simulink model "tempCyl4s"  (R2013a)
settings: Solver=ode15s  StartTime=0.0  StopTime=3  FixedStep=1e-3  RelTol=1e-5
values from neighbouring files (symbols this model uses):
  F0_ER = F_initial    [initHybrid.m]    (also in initMV.m; init_MVM.m)
  p0_AR = p_acool    [initHybrid.m]    (also in initMV.m; init_MVM.m)
  p0_ER = p_exh_init    [initHybrid.m]    (also in initMV.m; init_MVM.m)
  T0_AR = T_acool    [initHybrid.m]    (also in initMV.m; init_MVM.m)
  T0_ER = 800    [initHybrid.m]    (also in initMV.m; init_MVM.m)
  uGov = 0.2    [runTempCyl4S.m]
undefined symbols (not defined in the file): genset
libraries: EngineSystemSubmodelVer1_0 x6
settings Model: Creator=yum  LastModifiedBy=yum
settings DataIOCC: InspectSignalLogs=on

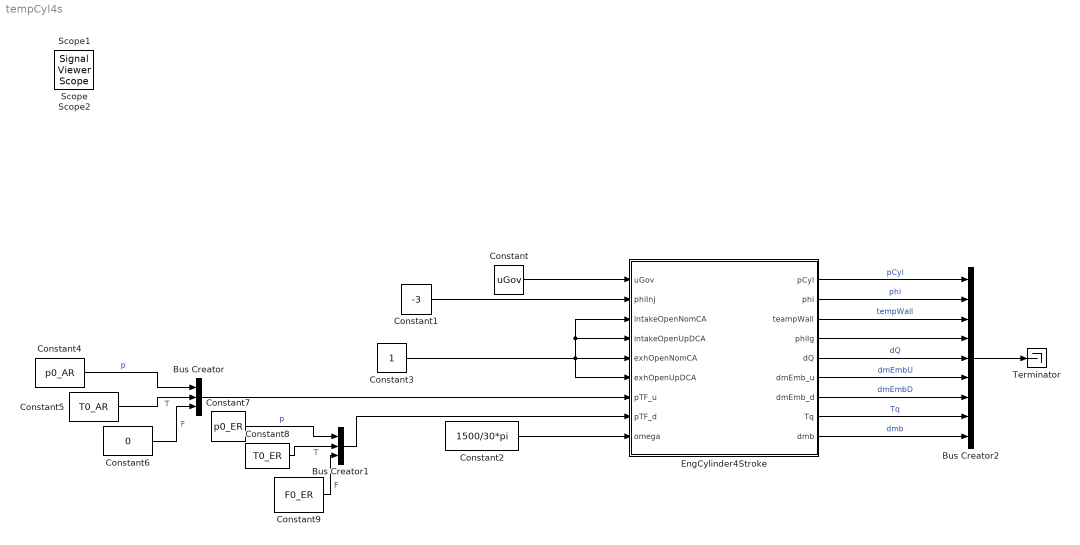
== system tempCyl4s ==
  Bus Creator : BusCreator  Inputs=3
  Bus Creator1 : BusCreator  Inputs=3
  Bus Creator2 : BusCreator  Inputs=9
  Constant : Constant  Value=uGov
  Constant1 : Constant  Value=-3
  Constant2 : Constant  Value=1500/30*pi
  Constant3 : Constant
  Constant4 : Constant  Value=p0_AR
  Constant5 : Constant  Value=T0_AR
  Constant6 : Constant  Value=0
  Constant7 : Constant  Value=p0_ER
  Constant8 : Constant  Value=T0_ER
  Constant9 : Constant  Value=F0_ER
  EngCylinder4Stroke : Subsystem  mask{fs=genset.eng.fs, nStroke=genset.eng.nStroke, hn=genset.eng.hn, nCyl=genset.eng.nCyl, iCyl=1, B=genset.eng.B, stroke=genset.eng.stroke, lambdaCrank=genset.eng.lambdaCrank, liftMaxIntake=genset.eng.intakeLiftMaxRef, DvIntake=genset.eng.intakeDV, betaIntake=genset.eng.intakeBeta, wIntake=genset.eng.intakeW, DpIntake=genset.eng.intakeDp, DsIntake=genset.eng.intakeDs, cAVVUpRef=genset.eng.cAVVUpRefIntake, cAVVDownRef=genset.eng.cAVVDownRefIntake, liftUpRef=genset.eng.liftUpRefIntake, liftDownRef=genset.eng.liftDownRefIntake, cAStartRef=genset.eng.startCARefIntake, dCALiftUp=genset.eng.dCALiftUpRefIntake, dCALiftDown=genset.eng.dCALiftDownIntake, dCALiftTopRef=genset.eng.dCALiftTopRefIntake, liftMaxExh=genset.eng.exhLiftMax, DvExh=genset.eng.exhDV, betaExh=genset.eng.exhBeta, wExh=genset.eng.exhW, DpExh=genset.eng.exhDp, DsExh=genset.eng.exhDs, cAVVUpRefExh=genset.eng.cAVVUpRefExh, cAVVDownRefExh=genset.eng.cAVVDownRefExh, liftUpRefExh=genset.eng.liftUpRefExh, liftDownRefExh=genset.eng.liftDownRefExh, cAStartRefExh=genset.eng.startCARefExh, dCALiftUpExh=genset.eng.dCALiftUpRefExh, dCALiftDownExh=genset.eng.dCALiftDownExh, dCALiftTopRefExh=genset.eng.dCALiftTopRefExh, mCp=genset.eng.mCp, cCylHT=genset.eng.cCylHT, cAlpha=genset.eng.cAlpha, mqfCycMax=genset.eng.mFCycMax, wiebePara=genset.eng.wiebePara, phi0=genset.eng.phi0, m0=genset.eng.mCyl0, E0=genset.eng.ECyl0, mb0=genset.eng.mbCyl0, V0=genset.eng.vCyl0, phi0A=genset.eng.phi0A, m0A=genset.eng.m0A, E0A=genset.eng.E0A, mb0A=genset.eng.mb0A, V0A=genset.eng.V0A}
      mask prompts: fs "Stoichiometric fuel-air ratio"; nStroke "Number of stroke"; hn "Lower heating value of the fuel [J/kg]"; nCyl "Number of cylinders"; iCyl "Cylinder number"; B "Bore of the cylinder [m]"; stroke "Stroke [m]"; lambdaCrank "Ratio of length of crank rod to connecting rod"; liftMaxIntake "Maximum valve lift [m]"; DvIntake "Valve head diameter [m]"; betaIntake "Seat angle [rad]"; wIntake "Valve seat width [m]"; DpIntake "Inner seat diameter [m]"; DsIntake "Stem diameter [m]"; cAVVUpRef "Crank angle array for opening [deg]"; cAVVDownRef "Crank angle array for closing [deg]"; liftUpRef "Normalized lift array for opening (0~1)"; liftDownRef "Normalized lift array for closing (0~1)"; cAStartRef "Nominal crank angle at start of valve lif [deg]"; dCALiftUp "Nominal duration of crank angle for valve opening [deg]"; dCALiftDown "Nominal duration of crank angle for valve closing [deg]"; dCALiftTopRef "Nominal duration of crank angle for valve open [deg]"; liftMaxExh "Maximum valve lift [m]"; DvExh "Valve head diameter [m]"; betaExh "Seat angle [rad]"; wExh "Valve seat width [m]"; DpExh "Inner seat diameter [m]"; DsExh "Stem diameter [m]"; cAVVUpRefExh "Crank angle array for opening [deg]"; cAVVDownRefExh "Crank angle array for closing [deg]"; liftUpRefExh "Normalized lift array for opening (0~1)"; liftDownRefExh "Normalized lift array for closing (0~1)"; cAStartRefExh "Nominal crank angle at start of valve lif [deg]"; dCALiftUpExh "Nominal duration of crank angle for valve opening [deg]"; dCALiftDownExh "Nominal duration of crank angle for valve closing [deg]"; dCALiftTopRefExh "Nominal duration of crank angle for valve open [deg]"; mCp "Heat capacity of the cylinder [J/K]"; cCylHT "Polynomial coefficient for heat rejection model from the cylinder (4 x 1)"; cAlpha "Fitting coefficient for convective heat transfer coefficient"; mqfCycMax "Maximum fuel mass injected per cycle [kg]"; wiebePara "3-Wiebe Parameters (9x1)"; phi0 "Initial crank angle [deg]"; m0 "Initial mass [kg]"; E0 "Initial internal energy [J]"; mb0 "Initial burned fuel mass [kg]"; V0 "Initial volume [m3]"; phi0A "Initial crank angle array [deg]"; m0A "Initial mass array [kg]"; E0A "Initial internal energy array [J]"; mb0A "Initial burned fuel mass array [kg]"; V0A "Initial volume array [m3]"
      mask init:
      | CylNo = uint8(iCyl);
      | if CylNo > 0 
      |     phi0 = phi0A(CylNo);
      |     m0 = m0A(CylNo);
      |     E0 = E0A(CylNo);
      |     mb0 = mb0A(CylNo);
      |     V0 = V0A(CylNo);
      | else
      |     phi0 = phi0A(1);
      |     m0 = m0A(1);
      |     E0 = E0A(1);
      |     mb0 = mb0A(1);
      |     V0 = V0A(1);
      | end;
      mask TypeOptions fs: ExhaustValve1/fs | IntakeValve1/fs | ThdynCV_VarVolNV/fs
      mask TypeOptions nStroke: ExhaustValve1/nStroke | IntakeValve1/nStroke | ROHR/nStroke
      mask TypeOptions hn: ROHR/hn
      mask TypeOptions nCyl: EngCylHeatTransfer/nCyl
      mask TypeOptions B: EngCylHeatTransfer/B | CrankMechKinematic1/B
      mask TypeOptions stroke: EngCylHeatTransfer/stroke | CrankMechKinematic1/stroke
      mask TypeOptions lambdaCrank: CrankMechKinematic1/lambdaCrank
      mask TypeOptions liftMaxIntake: IntakeValve1/liftMax
      mask TypeOptions DvIntake: IntakeValve1/Dv
      mask TypeOptions betaIntake: IntakeValve1/beta
      mask TypeOptions wIntake: IntakeValve1/w
      mask TypeOptions DpIntake: IntakeValve1/Dp
      mask TypeOptions DsIntake: IntakeValve1/Ds
      mask TypeOptions cAVVUpRef: IntakeValve1/cAVVUpRef
      mask TypeOptions cAVVDownRef: IntakeValve1/cAVVDownRef
      mask TypeOptions liftUpRef: IntakeValve1/liftUpRef
      mask TypeOptions liftDownRef: IntakeValve1/liftDownRef
      mask TypeOptions cAStartRef: IntakeValve1/cAStartRef
      mask TypeOptions dCALiftUp: IntakeValve1/dCALiftUp
      mask TypeOptions dCALiftDown: IntakeValve1/dCALiftDown
      mask TypeOptions dCALiftTopRef: IntakeValve1/dCALiftTopRef
      mask TypeOptions liftMaxExh: ExhaustValve1/liftMax
      mask TypeOptions DvExh: ExhaustValve1/Dv
      mask TypeOptions betaExh: ExhaustValve1/beta
      mask TypeOptions wExh: ExhaustValve1/w
      mask TypeOptions DpExh: ExhaustValve1/Dp
      mask TypeOptions DsExh: ExhaustValve1/Ds
      mask TypeOptions cAVVUpRefExh: ExhaustValve1/cAVVUpRef
      mask TypeOptions cAVVDownRefExh: ExhaustValve1/cAVVDownRef
      mask TypeOptions liftUpRefExh: ExhaustValve1/liftUpRef
      mask TypeOptions liftDownRefExh: ExhaustValve1/liftDownRef
      mask TypeOptions cAStartRefExh: ExhaustValve1/cAStartRef
      mask TypeOptions dCALiftUpExh: ExhaustValve1/dCALiftUp
      mask TypeOptions dCALiftDownExh: ExhaustValve1/dCALiftDown
      mask TypeOptions dCALiftTopRefExh: ExhaustValve1/dCALiftTopRef
      mask TypeOptions mCp: EngCylHeatTransfer/mCp
      mask TypeOptions cCylHT: EngCylHeatTransfer/cCylHT
      mask TypeOptions cAlpha: EngCylHeatTransfer/cAlpha
      mask TypeOptions mqfCycMax: ROHR/mqfCycMax
      mask TypeOptions wiebePara: ROHR/wiebePara
      mask TypeOptions phi0: CrankMechKinematic1/phi0
      mask TypeOptions m0: ThdynCV_VarVolNV/m0
      mask TypeOptions E0: ThdynCV_VarVolNV/E0
      mask TypeOptions mb0: ThdynCV_VarVolNV/mb0
      mask TypeOptions V0: ThdynCV_VarVolNV/V0
  Terminator : Terminator
  Scope : SignalViewerScope  IOType=viewer  ZoomMode=xonly  RefreshTime=0.035000
  Scope1 : SignalViewerScope  IOType=viewer  RefreshTime=0.035000
  Scope2 : SignalViewerScope  IOType=viewer  RefreshTime=0.035000
      settings: SaveName=ScopeData2
  wires:
  Constant/1 -> EngCylinder4Stroke/1(uGov)
  Constant1/1 -> EngCylinder4Stroke/2(phiInj)
  Constant2/1 -> EngCylinder4Stroke/9(omega)
  Constant3/1 -> EngCylinder4Stroke/3(intakeOpenNomCA), EngCylinder4Stroke/4(intakeOpenUpDCA), EngCylinder4Stroke/6(exhOpenUpDCA), EngCylinder4Stroke/5(exhOpenNomCA)
  Bus Creator/1 -> EngCylinder4Stroke/7(pTF_u)
  Constant4/1 -> Bus Creator/1  "p"
  Constant5/1 -> Bus Creator/2  "T"
  Constant6/1 -> Bus Creator/3  "F"
  Constant7/1 -> Bus Creator1/1  "p"
  Constant8/1 -> Bus Creator1/2  "T"
  Constant9/1 -> Bus Creator1/3  "F"
  Bus Creator1/1 -> EngCylinder4Stroke/8(pTF_d)
  EngCylinder4Stroke/2(phi) -> Bus Creator2/2  "phi"
  EngCylinder4Stroke/3(teampWall) -> Bus Creator2/3  "tempWall"
  EngCylinder4Stroke/1(pCyl) -> Bus Creator2/1  "pCyl"
  EngCylinder4Stroke/4(phiIg) -> Bus Creator2/4
  EngCylinder4Stroke/5(dQ) -> Bus Creator2/5  "dQ"
  EngCylinder4Stroke/6(dmEmb_u) -> Bus Creator2/6  "dmEmbU"
  EngCylinder4Stroke/7(dmEmb_d) -> Bus Creator2/7  "dmEmbD"
  EngCylinder4Stroke/8(Tq) -> Bus Creator2/8  "Tq"
  EngCylinder4Stroke/9(dmb) -> Bus Creator2/9  "dmb"
  Bus Creator2/1 -> Terminator/1

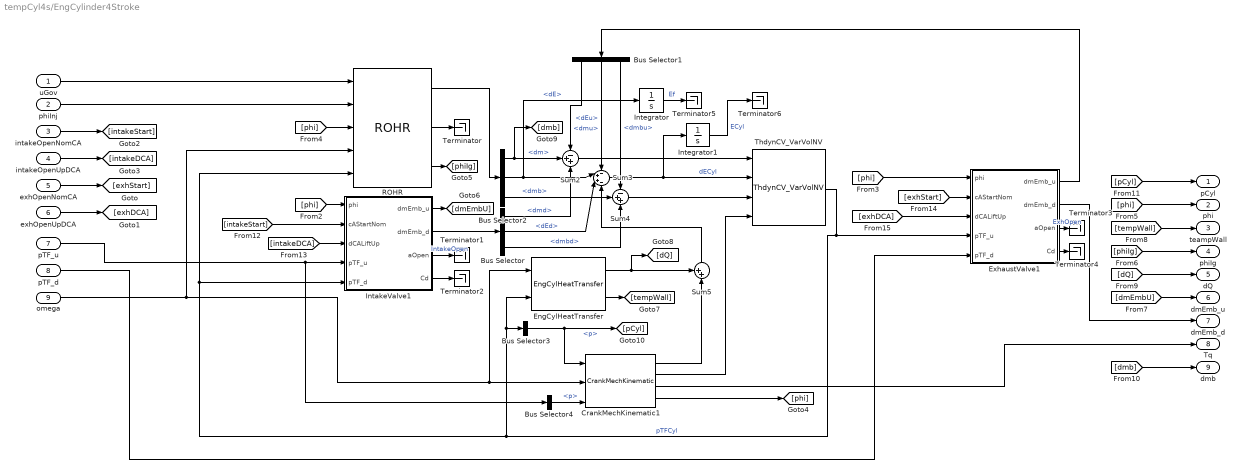
== system tempCyl4s/EngCylinder4Stroke ==
  uGov : Inport
  phiInj : Inport  Port=2
  intakeOpenNomCA : Inport  Port=3
  intakeOpenUpDCA : Inport  Port=4
  exhOpenNomCA : Inport  Port=5
  exhOpenUpDCA : Inport  Port=6
  pTF_u : Inport  Port=7
  pTF_d : Inport  Port=8
  omega : Inport  Port=9
  Bus Selector : BusSelector  OutputSignals=dmd,dEd,dmbd
  Bus Selector1 : BusSelector  OutputSignals=dmu,dEu,dmbu
  Bus Selector2 : BusSelector  OutputSignals=dm,dE,dmb
  Bus Selector3 : BusSelector  OutputSignals=p
  Bus Selector4 : BusSelector  OutputSignals=p
  CrankMechKinematic1 : EngineSystemSubmodelVer1_0/CrankMechKinematic  phi0=phi0  B=B  stroke=stroke  lambdaCrank=lambdaCrank
  EngCylHeatTransfer : EngineSystemSubmodelVer1_0/EngCylHeatTransfer  stroke=stroke  B=B  cAlpha=cAlpha  mCp=mCp  cCylHT=cCylHT  nCyl=nCyl  tempWall0=700
  ExhaustValve1 : Subsystem  mask{fs=fs, nStroke=nStroke, cAVVUpRef=cAVVUpRefExh, cAVVDownRef=cAVVDownRefExh, liftUpRef=liftUpRefExh, liftDownRef=liftDownRefExh, cAStartRef=cAStartRefExh, dCALiftUp=dCALiftUpExh, dCALiftDown=dCALiftDownExh, dCALiftTopRef=dCALiftTopRefExh, liftMax=liftMaxExh, Dv=DvExh, beta=betaExh, w=wExh, Dp=DpExh, Ds=DsExh}
      mask prompts: fs "Stoichiometric fuel-air equivalent ratio"; nStroke "Number of stroke"; cAVVUpRef "Crank angle array for opening [deg]"; cAVVDownRef "Crank angle array for closing [deg]"; liftUpRef "Normalized lift array for opening (0~1)"; liftDownRef "Normalized lift array for closing (0~1)"; cAStartRef "Nominal crank angle at start of valve lif [deg]"; dCALiftUp "Nominal duration of crank angle for valve opening [deg]"; dCALiftDown "Nominal duration of crank angle for valve closing [deg]"; dCALiftTopRef "Nominal duration of crank angle for valve open [deg]"; liftMax "Maximum valve lift [m]"; Dv "Valve head diameter [m]"; beta "Seat angle [rad]"; w "Valve seat width [m]"; Dp "Inner seat diameter [m]"; Ds "Stem diameter [m]"
      mask TypeOptions fs: IdealNozzle/fs
      mask TypeOptions nStroke: S-Function/nStroke
      mask TypeOptions cAVVUpRef: S-Function/cAVVUpRef
      mask TypeOptions cAVVDownRef: S-Function/cAVVDownRef
      mask TypeOptions liftUpRef: S-Function/liftUpRef
      mask TypeOptions liftDownRef: S-Function/liftDownRef
      mask TypeOptions cAStartRef: S-Function/cAStartRef
      mask TypeOptions dCALiftUp: S-Function/dCALiftUp
      mask TypeOptions dCALiftDown: S-Function/dCALiftDown
      mask TypeOptions dCALiftTopRef: S-Function/dCALiftTopRef
      mask TypeOptions liftMax: S-Function/liftMax
      mask TypeOptions Dv: S-Function1/Dv
      mask TypeOptions beta: S-Function1/beta
      mask TypeOptions w: S-Function1/w
      mask TypeOptions Dp: S-Function1/Dp
      mask TypeOptions Ds: S-Function1/Ds
  IntakeValve1 : Subsystem  mask{fs=fs, nStroke=nStroke, cAVVUpRef=cAVVUpRef, cAVVDownRef=cAVVDownRef, liftUpRef=liftUpRef, liftDownRef=liftDownRef, cAStartRef=cAStartRef, dCALiftUp=dCALiftUp, dCALiftDown=dCALiftDown, dCALiftTopRef=dCALiftTopRef, liftMax=liftMaxIntake, Dv=DvIntake, beta=betaIntake, w=wIntake, Dp=DpIntake, Ds=DsIntake}
      mask prompts: fs "Stoichiometric fuel-air equivalent ratio"; nStroke "Number of stroke"; cAVVUpRef "Crank angle array for opening [deg]"; cAVVDownRef "Crank angle array for closing [deg]"; liftUpRef "Normalized lift array for opening (0~1)"; liftDownRef "Normalized lift array for closing (0~1)"; cAStartRef "Nominal crank angle at start of valve lif [deg]"; dCALiftUp "Nominal duration of crank angle for valve opening [deg]"; dCALiftDown "Nominal duration of crank angle for valve closing [deg]"; dCALiftTopRef "Nominal duration of crank angle for valve open [deg]"; liftMax "Maximum valve lift [m]"; Dv "Valve head diameter [m]"; beta "Seat angle [rad]"; w "Valve seat width [m]"; Dp "Inner seat diameter [m]"; Ds "Stem diameter [m]"
      mask TypeOptions fs: IdealNozzle/fs
      mask TypeOptions nStroke: S-Function/nStroke
      mask TypeOptions cAVVUpRef: S-Function/cAVVUpRef
      mask TypeOptions cAVVDownRef: S-Function/cAVVDownRef
      mask TypeOptions liftUpRef: S-Function/liftUpRef
      mask TypeOptions liftDownRef: S-Function/liftDownRef
      mask TypeOptions cAStartRef: S-Function/cAStartRef
      mask TypeOptions dCALiftUp: S-Function/dCALiftUp
      mask TypeOptions dCALiftDown: S-Function/dCALiftDown
      mask TypeOptions dCALiftTopRef: S-Function/dCALiftTopRef
      mask TypeOptions liftMax: S-Function/liftMax
      mask TypeOptions Dv: S-Function1/Dv
      mask TypeOptions beta: S-Function1/beta
      mask TypeOptions w: S-Function1/w
      mask TypeOptions Dp: S-Function1/Dp
      mask TypeOptions Ds: S-Function1/Ds
  Integrator : Integrator
  Integrator1 : Integrator
  ROHR : EngineSystemSubmodelVer1_0/ROHR  mqfCycMax=mqfCycMax  wiebePara=wiebePara  hn=hn  nStroke=nStroke
  Sum2 : Sum  Inputs=-++
  Sum3 : Sum  Inputs=-++-
  Sum4 : Sum  Inputs=-++
  Sum5 : Sum  Inputs=++|
  Terminator{,1..6} (7 alike) : Terminator
  ThdynCV_VarVolNV : EngineSystemSubmodelVer1_0/ThdynCV_VarVolNV  fs=fs  m0=m0  E0=E0  mb0=mb0  V0=V0
  pCyl : Outport
  phi : Outport  Port=2
  teampWall : Outport  Port=3
  phiIg : Outport  Port=4
  dQ : Outport  Port=5
  dmEmb_u : Outport  Port=6
  dmEmb_d : Outport  Port=7
  Tq : Outport  Port=8
  dmb : Outport  Port=9
  wires:
  IntakeValve1/2(dmEmb_d) -> Bus Selector/1
  Sum2/1 -> ThdynCV_VarVolNV/1
  Sum3/1 -> Integrator1/1, ThdynCV_VarVolNV/2  "dECyl"
  Sum4/1 -> ThdynCV_VarVolNV/3
  ExhaustValve1/1(dmEmb_u) -> Bus Selector1/1
  Bus Selector1/1 -> Sum2/1  "<dmu>"
  Bus Selector1/2 -> Sum3/1  "<dEu>"
  Bus Selector1/3 -> Sum4/1  "<dmbu>"
  ThdynCV_VarVolNV/1 -> ROHR/5, IntakeValve1/5(pTF_d), Bus Selector3/1, EngCylHeatTransfer/2, ExhaustValve1/4(pTF_u)  "pTFCyl"
  Bus Selector/1 -> Sum2/3  "<dmd>"
  ROHR/1 -> Bus Selector2/1
  Bus Selector2/1 -> [dmb], Sum2/2  "<dm>"
  Bus Selector/2 -> Sum3/3  "<dEd>"
  Bus Selector/3 -> Sum4/3  "<dmbd>"
  Bus Selector2/3 -> Sum4/2  "<dmb>"
  omega/1 -> ROHR/4, EngCylHeatTransfer/1, CrankMechKinematic1/2
  Bus Selector3/1 -> [pCyl], CrankMechKinematic1/1  "<p>"
  CrankMechKinematic1/2 -> ThdynCV_VarVolNV/4
  CrankMechKinematic1/1 -> Sum5/2
  EngCylHeatTransfer/1 -> [dQ], Sum5/1
  CrankMechKinematic1/4 -> [phi]
  [phi] -> IntakeValve1/1(phi)
  [phi] -> ExhaustValve1/1(phi)
  pTF_u/1 -> Bus Selector4/1, IntakeValve1/4(pTF_u)
  Bus Selector4/1 -> CrankMechKinematic1/3  "<p>"
  pTF_d/1 -> ExhaustValve1/5(pTF_d)
  intakeOpenNomCA/1 -> [intakeStart]
  intakeOpenUpDCA/1 -> [intakeDCA]
  exhOpenNomCA/1 -> [exhStart]
  exhOpenUpDCA/1 -> [exhDCA]
  uGov/1 -> ROHR/1
  phiInj/1 -> ROHR/2
  [phi] -> ROHR/3
  ROHR/3 -> [phiIg]
  [phiIg] -> phiIg/1
  [phi] -> phi/1
  IntakeValve1/1(dmEmb_u) -> [dmEmbU]
  [dmEmbU] -> dmEmb_u/1
  ExhaustValve1/2(dmEmb_d) -> dmEmb_d/1
  EngCylHeatTransfer/2 -> [tempWall]
  [tempWall] -> teampWall/1
  [dQ] -> dQ/1
  CrankMechKinematic1/3 -> Tq/1
  [dmb] -> dmb/1
  [pCyl] -> pCyl/1
  [intakeStart] -> IntakeValve1/2(cAStartNom)
  [intakeDCA] -> IntakeValve1/3(dCALiftUp)
  [exhStart] -> ExhaustValve1/2(cAStartNom)
  [exhDCA] -> ExhaustValve1/3(dCALiftUp)
  ROHR/2 -> Terminator/1
  IntakeValve1/3(aOpen) -> Terminator1/1  "IntakeOpen"
  IntakeValve1/4(Cd) -> Terminator2/1
  ExhaustValve1/3(aOpen) -> Terminator3/1  "ExhOpen"
  ExhaustValve1/4(Cd) -> Terminator4/1
  Sum5/1 -> Sum3/4
  Bus Selector2/2 -> Sum3/2, Integrator/1  "<dE>"
  Integrator/1 -> Terminator5/1  "Ef"
  Integrator1/1 -> Terminator6/1  "ECyl"

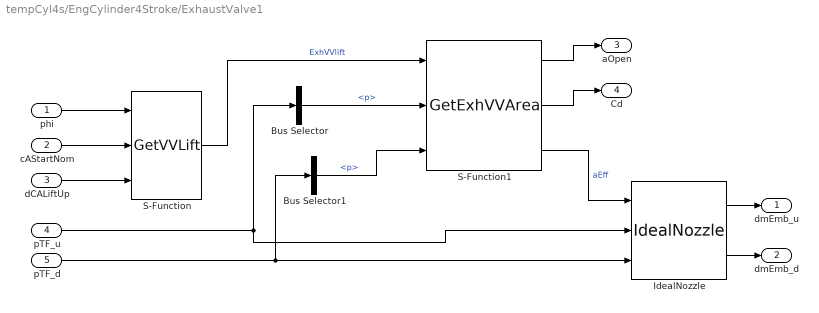
== system tempCyl4s/EngCylinder4Stroke/ExhaustValve1 ==
  phi : Inport
  cAStartNom : Inport  Port=2
  dCALiftUp : Inport  Port=3
  pTF_u : Inport  Port=4
  pTF_d : Inport  Port=5
  Bus Selector : BusSelector  OutputSignals=p
  Bus Selector1 : BusSelector  OutputSignals=p
  IdealNozzle : EngineSystemSubmodelVer1_0/IdealNozzle  fs=fs
  S-Function : S-Function  FunctionName=GetVVLift  Parameters=nStroke,liftMax,cAStartRef,dCALiftUp,dCALiftDown,dCALiftTopRef,cAVVUpRef,cAVVDownRef,liftUpRef,liftDownRef  EnableBusSupport=off  mask{nStroke=nStroke, liftMax=liftMax, cAStartRef=cAStartRef, dCALiftUp=dCALiftUp, dCALiftDown=dCALiftDown, dCALiftTopRef=dCALiftTopRef, cAVVUpRef=cAVVUpRef, cAVVDownRef=cAVVDownRef, liftUpRef=liftUpRef, liftDownRef=liftDownRef}
      mask prompts: nStroke "Number of stroke"; liftMax "Maximum valve lift [m]"; cAStartRef "Crank angle at the beginning of valve lift [deg]"; dCALiftUp "Duration for valve lifting [deg]"; dCALiftDown "Duration for valve closing [deg]"; dCALiftTopRef "Duration for valve fully opened [deg]"; cAVVUpRef "Crank angle array reference for valve opening [deg]"; cAVVDownRef "Crank angle array reference for valve closing [deg]"; liftUpRef "Normalized lift reference for valve opening (0~1)"; liftDownRef "Normalized lift reference for valve closing (0~1)"
  S-Function1 : S-Function  FunctionName=GetExhVVArea  Parameters=Dv,beta,w,Dp,Ds,coeffCdCorrP,coeffCdCorrQ,coeffCdCorrPR  EnableBusSupport=off  mask{Dv=Dv, beta=beta, w=w, Dp=Dp, Ds=Ds, coeffCdCorrP=[0.5329;-0.2047;0.04292], coeffCdCorrQ=[0.5359;-0.2962;0.06275], coeffCdCorrPR=[-0.006345;0.09503;0.8117]}
      mask prompts: Dv "Valve head diameter"; beta "Seat angle"; w "Valve seat width"; Dp "Inner seat diameter"; Ds "Stem diameter"; coeffCdCorrP "Produt coefficient for discharge coefficient for lift ratio"; coeffCdCorrQ "Quotient coefficient for discharge coefficient for lift ratio"; coeffCdCorrPR "Coefficient for discharge coefficient for pressure ratio"
  dmEmb_u : Outport
  dmEmb_d : Outport  Port=2
  aOpen : Outport  Port=3
  Cd : Outport  Port=4
  wires:
  S-Function1/2 -> Cd/1
  S-Function1/1 -> aOpen/1
  S-Function1/3 -> IdealNozzle/1  "aEff"
  dCALiftUp/1 -> S-Function/3
  cAStartNom/1 -> S-Function/2
  phi/1 -> S-Function/1
  IdealNozzle/1 -> dmEmb_u/1
  IdealNozzle/2 -> dmEmb_d/1
  pTF_u/1 -> IdealNozzle/2, Bus Selector/1
  pTF_d/1 -> Bus Selector1/1, IdealNozzle/3
  S-Function/1 -> S-Function1/1  "ExhVVlift"
  Bus Selector/1 -> S-Function1/2  "<p>"
  Bus Selector1/1 -> S-Function1/3  "<p>"

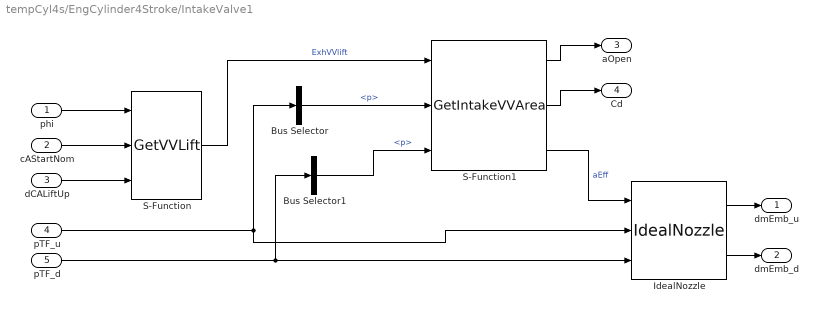
== system tempCyl4s/EngCylinder4Stroke/IntakeValve1 ==
  phi : Inport
  cAStartNom : Inport  Port=2
  dCALiftUp : Inport  Port=3
  pTF_u : Inport  Port=4
  pTF_d : Inport  Port=5
  Bus Selector : BusSelector  OutputSignals=p
  Bus Selector1 : BusSelector  OutputSignals=p
  IdealNozzle : EngineSystemSubmodelVer1_0/IdealNozzle  fs=fs
  S-Function : S-Function  FunctionName=GetVVLift  Parameters=nStroke,liftMax,cAStartRef,dCALiftUp,dCALiftDown,dCALiftTopRef,cAVVUpRef,cAVVDownRef,liftUpRef,liftDownRef  EnableBusSupport=off  mask{nStroke=nStroke, liftMax=liftMax, cAStartRef=cAStartRef, dCALiftUp=dCALiftUp, dCALiftDown=dCALiftDown, dCALiftTopRef=dCALiftTopRef, cAVVUpRef=cAVVUpRef, cAVVDownRef=cAVVDownRef, liftUpRef=liftUpRef, liftDownRef=liftDownRef}
      mask prompts: nStroke "Number of stroke"; liftMax "Maximum valve lift [m]"; cAStartRef "Crank angle at the beginning of valve lift [deg]"; dCALiftUp "Duration for valve lifting [deg]"; dCALiftDown "Duration for valve closing [deg]"; dCALiftTopRef "Duration for valve fully opened [deg]"; cAVVUpRef "Crank angle array reference for valve opening [deg]"; cAVVDownRef "Crank angle array reference for valve closing [deg]"; liftUpRef "Normalized lift reference for valve opening (0~1)"; liftDownRef "Normalized lift reference for valve closing (0~1)"
  S-Function1 : S-Function  FunctionName=GetIntakeVVArea  Parameters=Dv,beta,w,Dp,Ds  EnableBusSupport=off  mask{Dv=Dv, beta=beta, w=w, Dp=Dp, Ds=Ds}
      mask prompts: Dv "Valve head diameter"; beta "Seat angle"; w "Valve seat width"; Dp "Inner seat diameter"; Ds "Stem diameter"
  dmEmb_u : Outport
  dmEmb_d : Outport  Port=2
  aOpen : Outport  Port=3
  Cd : Outport  Port=4
  wires:
  S-Function1/2 -> Cd/1
  S-Function1/1 -> aOpen/1
  S-Function1/3 -> IdealNozzle/1  "aEff"
  dCALiftUp/1 -> S-Function/3
  cAStartNom/1 -> S-Function/2
  phi/1 -> S-Function/1
  IdealNozzle/1 -> dmEmb_u/1
  IdealNozzle/2 -> dmEmb_d/1
  pTF_u/1 -> IdealNozzle/2, Bus Selector/1
  pTF_d/1 -> Bus Selector1/1, IdealNozzle/3
  S-Function/1 -> S-Function1/1  "ExhVVlift"
  Bus Selector/1 -> S-Function1/2  "<p>"
  Bus Selector1/1 -> S-Function1/3  "<p>"
